simulink model "fuzzy_model"  (R2021a)
settings: Solver=VariableStepAuto  StartTime=0.0  StopTime=5  RelTol=1e-3
libraries: fuzblock x2, pid_lib x2
settings Model: Creator=hty  LastModifiedBy=hty

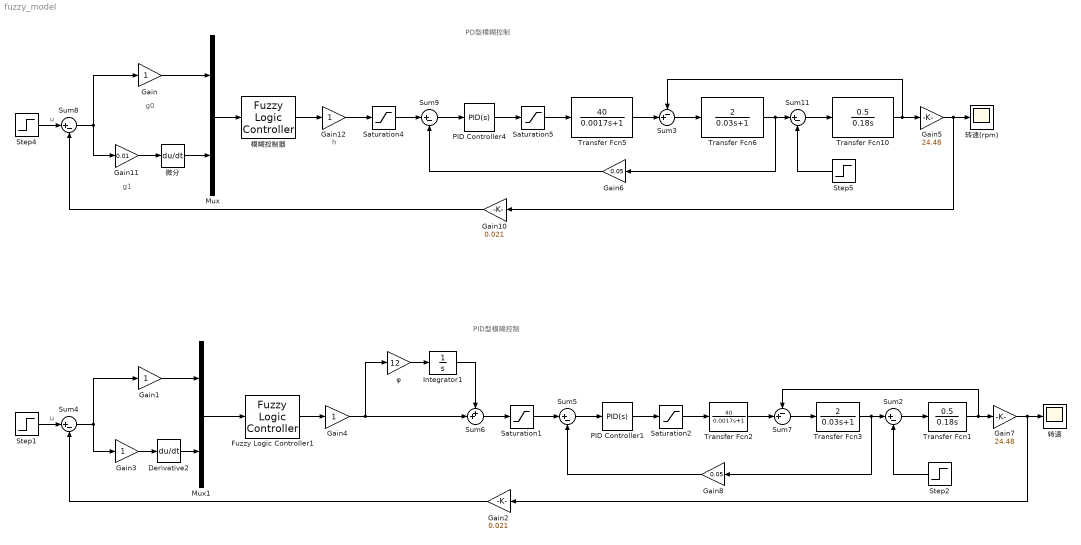
== system fuzzy_model ==
  note: PID型模糊控制
  note: PD型模糊控制
  note: h
  note: g1
  note: g0
  note: u
  note: u
  Derivative2 : Derivative
  Fuzzy Logic Controller1 : fuzblock/Fuzzy Logic  Controller  FIS='fuzzy_controller.fis'  OutputSampleNumber=101  DataType=double  FuzzifiedInputs=off  RuleFiringStrengths=off  RuleOutputs=off  AggregatedOutputs=off  SimulateUsing=Interpreted execution  OutOfRangeInputValueMessage=warning  NoRuleFiredMessage=warning  EmptyOutputFuzzySetMessage=warning
  Gain{,1,3..4,12} (5 alike) : Gain
  Gain10 : Gain  Gain=0.021
  Gain11 : Gain  Gain=0.01
  Gain2 : Gain  Gain=0.021
  Gain5 : Gain  Gain=24.48
  Gain6 : Gain  Gain=0.05
  Gain7 : Gain  Gain=24.48
  Gain8 : Gain  Gain=0.05
  Integrator1 : Integrator  UpperSaturationLimit=0.1  LowerSaturationLimit=-0.1
  Mux : Mux  Inputs=2
  Mux1 : Mux  Inputs=2
  PID Controller1 : pid_lib/PID Controller  Controller=PID  Form=Parallel  TimeDomain=Continuous-time  UseExternalTs=off  SampleTime=-1  IntegratorMethod=Forward Euler  FilterMethod=Forward Euler  ControllerParametersSource=internal  P=1.013  I=34.8  D=0  UseFilter=on  N=100  TunerSelectOption=Transfer Function Based (PID Tuner App)  InitialConditionSource=internal  InitialConditionForIntegrator=0  InitialConditionForFilter=0  DifferentiatorICPrevScaledInput=0  ExternalReset=none  TrackingMode=off  Kt=1  LimitOutput=off  SatLimitsSource=internal  UpperSaturationLimit=inf  LowerSaturationLimit=-inf  LinearizeAsGain=on  AntiWindupMode=none  Kb=1  POutMin=[]  POutMax=[]  IOutMin=[]  IOutMax=[]  DOutMin=[]  DOutMax=[]  NOutMin=[]  NOutMax=[]  SumOutMin=[]  SumOutMax=[]  SaturationOutMin=[]  SaturationOutMax=[]  PParamMin=[]  PParamMax=[]  IParamMin=[]  IParamMax=[]  DParamMin=[]  DParamMax=[]  NParamMin=[]  NParamMax=[]  KbParamMin=[]  KbParamMax=[]  KtParamMin=[]  KtParamMax=[]  KbOutMin=[]  KbOutMax=[]  KtOutMin=[]  KtOutMax=[]  IntegratorOutMin=[]  IntegratorOutMax=[]  FilterOutMin=[]  FilterOutMax=[]  SumI1OutMin=[]  SumI1OutMax=[]  SumI2OutMin=[]  SumI2OutMax=[]  SumI3OutMin=[]  SumI3OutMax=[]  SumI4OutMin=[]  SumI4OutMax=[]  SumDOutMin=[]  SumDOutMax=[]  DifferentiatorOutMin=[]  DifferentiatorOutMax=[]  FilterDiffOutCoefMin=[]  FilterDiffOutCoefMax=[]  ReciprocalOutMin=[]  ReciprocalOutMax=[]  SumDenOutMin=[]  SumDenOutMax=[]  SumNumOutMin=[]  SumNumOutMax=[]  DivideOutMin=[]  DivideOutMax=[]  UdiffTsProdOutMin=[]  UdiffTsProdOutMax=[]  NTsProdOutMin=[]  NTsProdOutMax=[]  UintegralTsProdOutMin=[]  UintegralTsProdOutMax=[]  UngainTsProdOutMin=[]  UngainTsProdOutMax=[]  IntegratorContinuousStateAttributes=''  IntegratorStateMustResolveToSignalObject=off  IntegratorRTWStateStorageClass=Auto  FilterContinuousStateAttributes=''  FilterStateMustResolveToSignalObject=off  FilterRTWStateStorageClass=Auto  ParallelPVariant=InternalParameters  IdealPVariant=Disabled  IVariant=InternalParameters  DVariant=InternalParameters  IntegratorVariant=Continuous  SatVariant=Disabled  AWVariant=Passthrough  PCopyVariant=Disabled  TRVariant=Disabled  FdbkBlocksVariant=Forward  IdealPFdbkVariant=Disabled  SatFdbkVariant=Disabled  DerivativeFilterVariant=ContFilter  NVariant=InternalParameters  NCopyVariant=Disabled  FilterICVariant=InternalICsFilter  IntegratorICVariant=InternalICs  ExternalResetVariant=Disabled  TRSumVariant=Passthrough  SumFdbkVariant=Disabled  SumVariant=Sum_PID  TsampFilterVariant=InternalTs  TsampNgainVariant=Passthrough  TsampIntegralVariant=Passthrough  ExternalSaturationOutDataTypeStr=Inherit: Same as second input
  PID Controller4 : pid_lib/PID Controller  Controller=PID  Form=Parallel  TimeDomain=Continuous-time  UseExternalTs=off  SampleTime=-1  IntegratorMethod=Forward Euler  FilterMethod=Forward Euler  ControllerParametersSource=internal  P=1.013  I=34.8  D=0  UseFilter=on  N=100  TunerSelectOption=Transfer Function Based (PID Tuner App)  InitialConditionSource=internal  InitialConditionForIntegrator=0  InitialConditionForFilter=0  DifferentiatorICPrevScaledInput=0  ExternalReset=none  TrackingMode=off  Kt=1  LimitOutput=off  SatLimitsSource=internal  UpperSaturationLimit=inf  LowerSaturationLimit=-inf  LinearizeAsGain=on  AntiWindupMode=none  Kb=1  POutMin=[]  POutMax=[]  IOutMin=[]  IOutMax=[]  DOutMin=[]  DOutMax=[]  NOutMin=[]  NOutMax=[]  SumOutMin=[]  SumOutMax=[]  SaturationOutMin=[]  SaturationOutMax=[]  PParamMin=[]  PParamMax=[]  IParamMin=[]  IParamMax=[]  DParamMin=[]  DParamMax=[]  NParamMin=[]  NParamMax=[]  KbParamMin=[]  KbParamMax=[]  KtParamMin=[]  KtParamMax=[]  KbOutMin=[]  KbOutMax=[]  KtOutMin=[]  KtOutMax=[]  IntegratorOutMin=[]  IntegratorOutMax=[]  FilterOutMin=[]  FilterOutMax=[]  SumI1OutMin=[]  SumI1OutMax=[]  SumI2OutMin=[]  SumI2OutMax=[]  SumI3OutMin=[]  SumI3OutMax=[]  SumI4OutMin=[]  SumI4OutMax=[]  SumDOutMin=[]  SumDOutMax=[]  DifferentiatorOutMin=[]  DifferentiatorOutMax=[]  FilterDiffOutCoefMin=[]  FilterDiffOutCoefMax=[]  ReciprocalOutMin=[]  ReciprocalOutMax=[]  SumDenOutMin=[]  SumDenOutMax=[]  SumNumOutMin=[]  SumNumOutMax=[]  DivideOutMin=[]  DivideOutMax=[]  UdiffTsProdOutMin=[]  UdiffTsProdOutMax=[]  NTsProdOutMin=[]  NTsProdOutMax=[]  UintegralTsProdOutMin=[]  UintegralTsProdOutMax=[]  UngainTsProdOutMin=[]  UngainTsProdOutMax=[]  IntegratorContinuousStateAttributes=''  IntegratorStateMustResolveToSignalObject=off  IntegratorRTWStateStorageClass=Auto  FilterContinuousStateAttributes=''  FilterStateMustResolveToSignalObject=off  FilterRTWStateStorageClass=Auto  ParallelPVariant=InternalParameters  IdealPVariant=Disabled  IVariant=InternalParameters  DVariant=InternalParameters  IntegratorVariant=Continuous  SatVariant=Disabled  AWVariant=Passthrough  PCopyVariant=Disabled  TRVariant=Disabled  FdbkBlocksVariant=Forward  IdealPFdbkVariant=Disabled  SatFdbkVariant=Disabled  DerivativeFilterVariant=ContFilter  NVariant=InternalParameters  NCopyVariant=Disabled  FilterICVariant=InternalICsFilter  IntegratorICVariant=InternalICs  ExternalResetVariant=Disabled  TRSumVariant=Passthrough  SumFdbkVariant=Disabled  SumVariant=Sum_PID  TsampFilterVariant=InternalTs  TsampNgainVariant=Passthrough  TsampIntegralVariant=Passthrough  ExternalSaturationOutDataTypeStr=Inherit: Same as second input
  Saturation1 : Saturate  UpperLimit=200  LowerLimit=-200
  Saturation2 : Saturate  UpperLimit=100  LowerLimit=-100
  Saturation4 : Saturate  UpperLimit=200  LowerLimit=-200
  Saturation5 : Saturate  UpperLimit=100  LowerLimit=-100
  Step1 : Step  Time=0  After=10  SampleTime=0
  Step2 : Step  Time=2  After=10  SampleTime=0
  Step4 : Step  Time=0  After=10  SampleTime=0
  Step5 : Step  Time=2  After=10  SampleTime=0
  Sum{2,4..5,8..9,11} (6 alike) : Sum  Inputs=|+-
  Sum3 : Sum  Inputs=-+|
  Sum6 : Sum  Inputs=++|
  Sum7 : Sum  Inputs=-+|
  Transfer Fcn1 : TransferFcn  Numerator=0.5  Denominator=[0.18 0]
  Transfer Fcn10 : TransferFcn  Numerator=0.5  Denominator=[0.18 0]
  Transfer Fcn2 : TransferFcn  Numerator=40  Denominator=[0.0017 1]
  Transfer Fcn3 : TransferFcn  Numerator=2  Denominator=[0.03 1]
  Transfer Fcn5 : TransferFcn  Numerator=40  Denominator=[0.0017 1]
  Transfer Fcn6 : TransferFcn  Numerator=2  Denominator=[0.03 1]
  φ : Gain  Gain=12
  微分 : Derivative
  模糊控制器 : fuzblock/Fuzzy Logic  Controller  FIS='fuzzy_controller.fis'  OutputSampleNumber=101  DataType=double  FuzzifiedInputs=off  RuleFiringStrengths=off  RuleOutputs=off  AggregatedOutputs=off  SimulateUsing=Interpreted execution  OutOfRangeInputValueMessage=warning  NoRuleFiredMessage=warning  EmptyOutputFuzzySetMessage=warning
  转速 : Scope
  转速(rpm) : Scope
  wires:
  Transfer Fcn5/1 -> Sum3/2
  Sum9/1 -> PID Controller4/1
  Step4/1 -> Sum8/1
  Transfer Fcn10/1 -> Sum3/1, Gain5/1
  Sum3/1 -> Transfer Fcn6/1
  Gain11/1 -> 微分/1
  微分/1 -> Mux/2
  Saturation5/1 -> Transfer Fcn5/1
  模糊控制器/1 -> Gain12/1
  Gain5/1 -> 转速(rpm)/1, Gain10/1
  Gain10/1 -> Sum8/2
  Gain/1 -> Mux/1
  PID Controller4/1 -> Saturation5/1
  Gain12/1 -> Saturation4/1
  Sum11/1 -> Transfer Fcn10/1
  Saturation4/1 -> Sum9/1
  Gain6/1 -> Sum9/2
  Step5/1 -> Sum11/2
  Mux/1 -> 模糊控制器/1
  Transfer Fcn6/1 -> Sum11/1, Gain6/1
  Sum8/1 -> Gain11/1, Gain/1
  Sum5/1 -> PID Controller1/1
  Sum2/1 -> Transfer Fcn1/1
  Sum7/1 -> Transfer Fcn3/1
  Step1/1 -> Sum4/1
  Step2/1 -> Sum2/2
  PID Controller1/1 -> Saturation2/1
  Mux1/1 -> Fuzzy Logic Controller1/1
  Gain1/1 -> Mux1/1
  Gain7/1 -> 转速/1, Gain2/1
  Gain2/1 -> Sum4/2
  Derivative2/1 -> Mux1/2
  Transfer Fcn2/1 -> Sum7/2
  Sum4/1 -> Gain3/1, Gain1/1
  Gain3/1 -> Derivative2/1
  Saturation1/1 -> Sum5/1
  Gain8/1 -> Sum5/2
  Transfer Fcn1/1 -> Sum7/1, Gain7/1
  Saturation2/1 -> Transfer Fcn2/1
  Fuzzy Logic Controller1/1 -> Gain4/1
  Transfer Fcn3/1 -> Gain8/1, Sum2/1
  Sum6/1 -> Saturation1/1
  Gain4/1 -> φ/1, Sum6/2
  φ/1 -> Integrator1/1
  Integrator1/1 -> Sum6/1
